simulink model "MSIwS_2007_2008_L_T9_ekg"  (Simulink 6.6)
settings: Solver=ode45  StartTime=0.0  StopTime=t_sym  FixedStep=0.0001  RelTol=1e-3
values from neighbouring files (symbols this model uses):
  Ud = 5    [Lab4_zad2.m]
  Ug = 0.1    [Lab4_zad2.m]
libraries: simulink x4
settings Model: Creator=Praca  LastModifiedBy=Praca
settings DebuggingCC: SignalResolutionControl=TryResolveAllWithWarning  SolverPrmCheckMsg=none  MultiTaskDSMMsg=warning  MultiTaskCondExecSysMsg=none
settings RTWCC: IncludeERTFirstTime=on

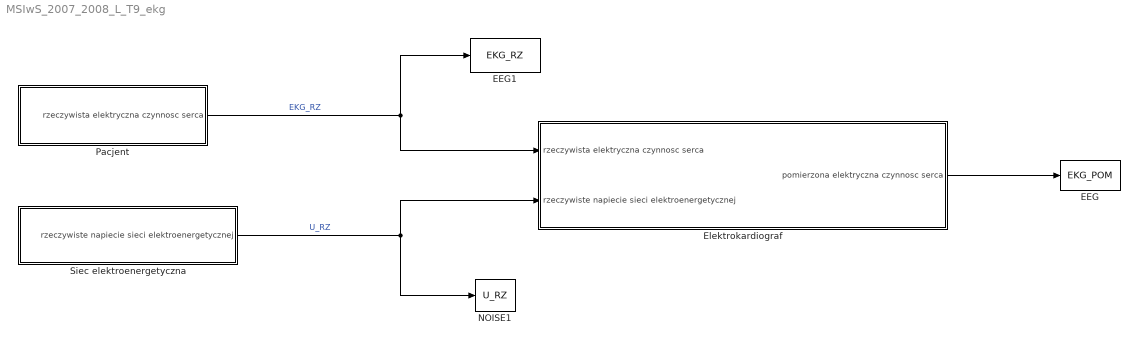
== system MSIwS_2007_2008_L_T9_ekg ==
  EEG : ToWorkspace  VariableName=EKG_POM  SampleTime=-1  SaveFormat=Array
  EEG1 : ToWorkspace  VariableName=EKG_RZ  SampleTime=-1  SaveFormat=Array
  Elektrokardiograf : Subsystem
  NOISE1 : ToWorkspace  VariableName=U_RZ  SampleTime=-1  SaveFormat=Array
  Pacjent : Subsystem
  Siec elektroenergetyczna : Subsystem
  wires:
  Pacjent/1(rzeczywista elektryczna czynnosc serca) -> EEG1/1, Elektrokardiograf/1(rzeczywista elektryczna czynnosc serca)  "EKG_RZ"
  Elektrokardiograf/1(pomierzona elektryczna czynnosc serca) -> EEG/1
  Siec elektroenergetyczna/1(rzeczywiste napiecie sieci elektroenergetycznej) -> NOISE1/1, Elektrokardiograf/2(rzeczywiste napiecie sieci elektroenergetycznej)  "U_RZ"

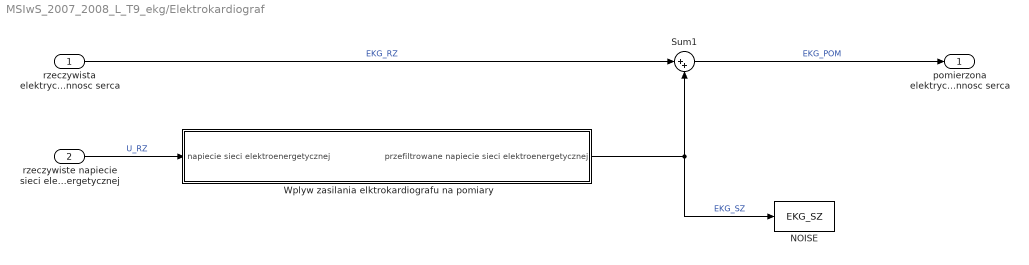
== system MSIwS_2007_2008_L_T9_ekg/Elektrokardiograf ==
  rzeczywista elektryczna czynnosc serca : Inport
  rzeczywiste napiecie sieci elektroenergetycznej : Inport  Port=2
  NOISE : ToWorkspace  VariableName=EKG_SZ  SampleTime=-1  SaveFormat=Array
  Sum1 : Sum  Inputs=|++
  Wplyw zasilania elktrokardiografu na pomiary : Subsystem
  pomierzona elektryczna czynnosc serca : Outport
  wires:
  Wplyw zasilania elktrokardiografu na pomiary/1(przefiltrowane napiecie sieci elektroenergetycznej) -> Sum1/2, NOISE/1  "EKG_SZ"
  rzeczywista elektryczna czynnosc serca/1 -> Sum1/1  "EKG_RZ"
  rzeczywiste napiecie sieci elektroenergetycznej/1 -> Wplyw zasilania elktrokardiografu na pomiary/1(napiecie sieci elektroenergetycznej)  "U_RZ"
  Sum1/1 -> pomierzona elektryczna czynnosc serca/1  "EKG_POM"

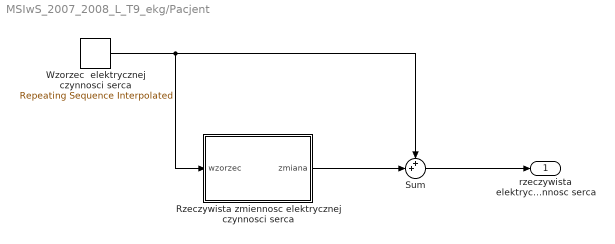
== system MSIwS_2007_2008_L_T9_ekg/Pacjent ==
  Rzeczywista zmiennosc elektrycznej czynnosci serca : Subsystem
  Sum : Sum  Inputs=++|
  Wzorzec  elektrycznej czynnosci serca : simulink/Sources/Repeating Sequence Interpolated  SystemSampleTime=-1  OutValues=[3 1 1.5 -7 20 1 0 -1 -2 0 4.5 4 4 4 4 4 4 4 4 4 5 ].'  TimeValues=1/40*[0 1 2 3 4 5 6 7 8 9 10 11 12 13 14 15 16 17 18 19 20].'  LookUpMeth=Interpolation-Use End Values  tsamp=0.001  OutputDataTypeScalingMode=Specify via dialog  OutDataType=float('double')  OutScaling=2^-10
  rzeczywista elektryczna czynnosc serca : Outport
  wires:
  Wzorzec  elektrycznej czynnosci serca/1 -> Sum/1, Rzeczywista zmiennosc elektrycznej czynnosci serca/1(wzorzec)
  Rzeczywista zmiennosc elektrycznej czynnosci serca/1(zmiana) -> Sum/2
  Sum/1 -> rzeczywista elektryczna czynnosc serca/1

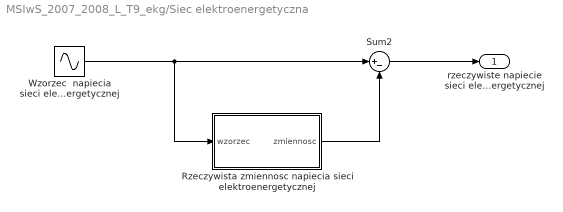
== system MSIwS_2007_2008_L_T9_ekg/Siec elektroenergetyczna ==
  Rzeczywista zmiennosc napiecia sieci elektroenergetycznej : Subsystem
  Sum2 : Sum  Inputs=|+-
  Wzorzec  napiecia sieci elektroenergetycznej : Sin  Amplitude=230  Frequency=314  SampleTime=0.001
  rzeczywiste napiecie sieci elektroenergetycznej : Outport
  wires:
  Wzorzec  napiecia sieci elektroenergetycznej/1 -> Rzeczywista zmiennosc napiecia sieci elektroenergetycznej/1(wzorzec), Sum2/1
  Sum2/1 -> rzeczywiste napiecie sieci elektroenergetycznej/1
  Rzeczywista zmiennosc napiecia sieci elektroenergetycznej/1(zmiennosc) -> Sum2/2

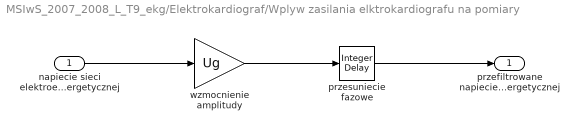
== system MSIwS_2007_2008_L_T9_ekg/Elektrokardiograf/Wplyw zasilania elktrokardiografu na pomiary ==
  napiecie sieci elektroenergetycznej : Inport
  przesuniecie fazowe : simulink/Discrete/Integer Delay  vinit=0.0  samptime=0.001  NumDelays=Ud
  wzmocnienie amplitudy : Gain  Gain=Ug  SampleTime=0.001
  przefiltrowane napiecie sieci elektroenergetycznej : Outport
  wires:
  wzmocnienie amplitudy/1 -> przesuniecie fazowe/1
  napiecie sieci elektroenergetycznej/1 -> wzmocnienie amplitudy/1
  przesuniecie fazowe/1 -> przefiltrowane napiecie sieci elektroenergetycznej/1

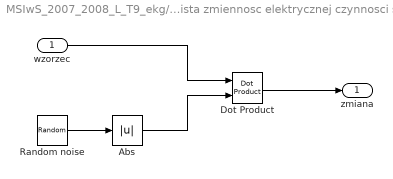
== system MSIwS_2007_2008_L_T9_ekg/Pacjent/Rzeczywista zmiennosc elektrycznej czynnosci serca ==
  wzorzec : Inport
  Abs : Abs  SampleTime=0.001
  Dot Product : simulink/Math Operations/Dot Product  InputSameDT=on  OutDataType=sfix(16)  OutScaling=2^-10  DoSatur=off
  Random noise : RandomNumber  Variance=0.0025  SampleTime=0.001*500
  zmiana : Outport
  wires:
  Abs/1 -> Dot Product/2
  Random noise/1 -> Abs/1
  wzorzec/1 -> Dot Product/1
  Dot Product/1 -> zmiana/1

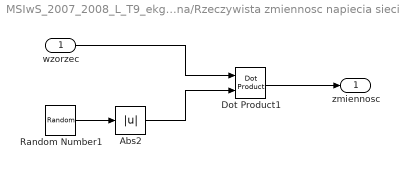
== system MSIwS_2007_2008_L_T9_ekg/Siec elektroenergetyczna/Rzeczywista zmiennosc napiecia sieci elektroenergetycznej ==
  wzorzec : Inport
  Abs2 : Abs  SampleTime=0.001
  Dot Product1 : simulink/Math Operations/Dot Product  InputSameDT=on  OutDataType=sfix(16)  OutScaling=2^-10  DoSatur=off
  Random Number1 : RandomNumber  Variance=0.0004  SampleTime=0.001*20
  zmiennosc : Outport
  wires:
  Random Number1/1 -> Abs2/1
  Dot Product1/1 -> zmiennosc/1
  Abs2/1 -> Dot Product1/2
  wzorzec/1 -> Dot Product1/1
